simulink model "MODEL_BicycleModel_Integrator_SS_and_TF"  (R2019b)
settings: Solver=ode45  StartTime=0.0  StopTime=500  MaxStep=0.01  RelTol=1e-3  EnableMultiTasking=on
values from neighbouring files (symbols this model uses):
  a = vehicle(i).a    [SCRIPT_BicycleModel_Integrator_SS_and_TF.m]
  A = [(Caf+Car)/(m*U) (a*Caf-b*Car)/(m*U)-U ... (first row only)    [SCRIPT_BicycleModel_Integrator_SS_and_TF.m]
  b = vehicle(i).b    [SCRIPT_BicycleModel_Integrator_SS_and_TF.m]
  B = [-Caf/m -Car/m; -a*Caf/Iz b*Car/Iz]    [SCRIPT_BicycleModel_Integrator_SS_and_TF.m]
  Caf = vehicle(i).Caf    [SCRIPT_BicycleModel_Integrator_SS_and_TF.m]
  Car = vehicle(i).Car    [SCRIPT_BicycleModel_Integrator_SS_and_TF.m]
  den = [1 -((Caf+Car)/(m*U)+(Caf*a^2+Car*b^2)/(Iz*U)) (Caf*Car*L^2/(m*Iz*U^2)+(a*Caf-b*Car)/Iz)]    [SCRIPT_BicycleModel_Integrator_SS_and_TF.m]
  Iz = vehicle(i).Iz    [SCRIPT_BicycleModel_Integrator_SS_and_TF.m]
  m = vehicle(i).m    [SCRIPT_BicycleModel_Integrator_SS_and_TF.m]
  num_latvel = [-Caf/m b*Caf*Car*L/(m*U*Iz)+a*Caf*U/Iz]    [SCRIPT_BicycleModel_Integrator_SS_and_TF.m]
  num_yawrate = [-a*Caf/Iz Caf*Car*L/(m*U*Iz)]    [SCRIPT_BicycleModel_Integrator_SS_and_TF.m]
  U = 20    [SCRIPT_BicycleModel_Integrator_SS_and_TF.m]
settings Model: Creator=snb10  LastModifiedBy=Dada
settings DataIOCC: LimitDataPoints=on  SaveFormat=Array  SignalLoggingSaveFormat=ModelDataLogs  ReturnWorkspaceOutputs=off  SignalLoggingName=sigsOut
settings OptimizationCC: InitFltsAndDblsToZero=on  LifeSpan=inf
settings DebuggingCC: SaveWithParameterizedLinksMsg=none  UnderspecifiedInitializationDetection=Classic  MergeDetectMultiDrivingBlocksExec=none  SignalResolutionControl=TryResolveAllWithWarning  MultiTaskDSMMsg=warning  MultiTaskCondExecSysMsg=none  FcnCallInpInsideContextMsg=warning  StateNameClashWarn=warning  SFUnexpectedBacktrackingDiag=warning  SFNoUnconditionalDefaultTransitionDiag=warning  SFExecutionAtInitializationDiag=none  ArithmeticOperatorsInVariantConditions=warning
settings HardwareCC: ProdBitPerPointer=32  ProdBitPerSizeT=32  ProdBitPerPtrDiffT=32  ProdLargestAtomicFloat=None  ProdIntDivRoundTo=Undefined  ProdEndianess=Unspecified  ProdWordSize=32  ProdHWDeviceType=32-bit Generic  TargetUnknown=on
settings ModelReferenceCC: PropagateSignalLabelsOutOfModel=off
settings SFSimCC: SimUseLocalCustomCode=off  CustomCodeUndefinedFunction=UseInterfaceOnly
settings RTWCC: RTWUseLocalCustomCode=off
settings CodeAppCC: StateflowObjectComments=on
settings GRTTargetCC: TargetFcnLib=ansi_tfl_tmw.mat  TargetLangStandard=C89/C90 (ANSI)  GeneratePreprocessorConditionals=Disable all  CombineOutputUpdateFcns=off  GRTInterface=on
settings ConfigComp: CovMetricSettings=dw  CovHtmlReporting=on  CovSaveCumulativeToWorkspaceVar=on  CovSaveSingleToWorkspaceVar=on  CovExternalEMLEnable=off

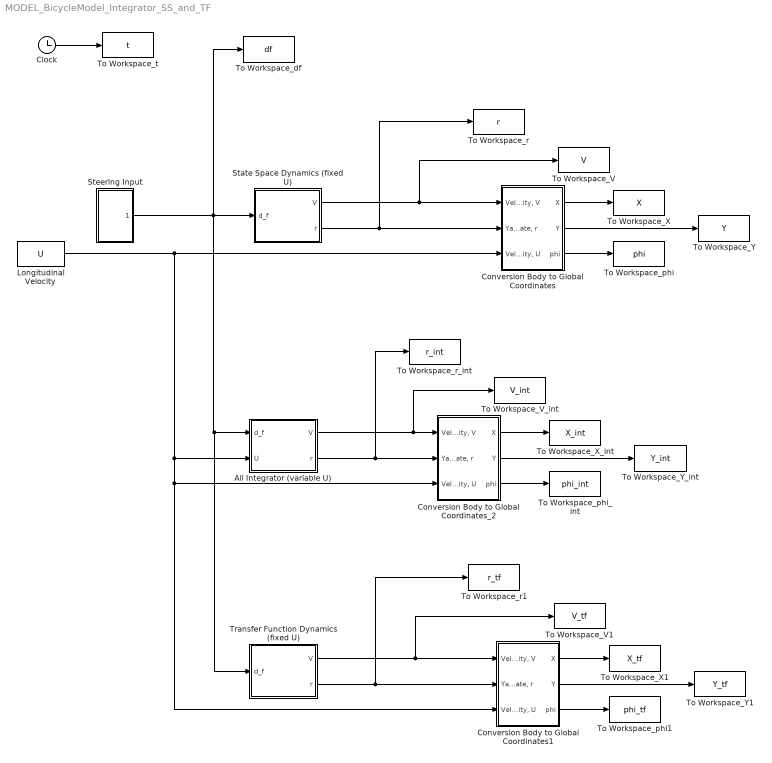
== system MODEL_BicycleModel_Integrator_SS_and_TF ==
  All Integrator (variable U) : Subsystem
  Clock : Clock
  Conversion Body to Global Coordinates : Subsystem
  Conversion Body to Global Coordinates1 : Subsystem
  Conversion Body to Global Coordinates_2 : Subsystem
  Longitudinal Velocity : Constant  Value=U
  State Space Dynamics (fixed U) : Subsystem
  Steering Input : Subsystem
  To Workspace_V : ToWorkspace  VariableName=V  SampleTime=-1
  To Workspace_V1 : ToWorkspace  VariableName=V_tf  SampleTime=-1
  To Workspace_V_int : ToWorkspace  VariableName=V_int  SampleTime=-1
  To Workspace_X : ToWorkspace  VariableName=X  SampleTime=-1
  To Workspace_X1 : ToWorkspace  VariableName=X_tf  SampleTime=-1
  To Workspace_X_int : ToWorkspace  VariableName=X_int  SampleTime=-1
  To Workspace_Y : ToWorkspace  VariableName=Y  SampleTime=-1
  To Workspace_Y1 : ToWorkspace  VariableName=Y_tf  SampleTime=-1
  To Workspace_Y_int : ToWorkspace  VariableName=Y_int  SampleTime=-1
  To Workspace_df : ToWorkspace  VariableName=df  SampleTime=-1
  To Workspace_phi : ToWorkspace  VariableName=phi  SampleTime=-1
  To Workspace_phi1 : ToWorkspace  VariableName=phi_tf  SampleTime=-1
  To Workspace_phi_int : ToWorkspace  VariableName=phi_int  SampleTime=-1
  To Workspace_r : ToWorkspace  VariableName=r  SampleTime=-1
  To Workspace_r1 : ToWorkspace  VariableName=r_tf  SampleTime=-1
  To Workspace_r_int : ToWorkspace  VariableName=r_int  SampleTime=-1
  To Workspace_t : ToWorkspace  VariableName=t  SampleTime=-1
  Transfer Function Dynamics (fixed U) : Subsystem
  wires:
  Conversion Body to Global Coordinates/1(X) -> To Workspace_X/1
  Conversion Body to Global Coordinates/2(Y) -> To Workspace_Y/1
  Conversion Body to Global Coordinates/3(phi) -> To Workspace_phi/1
  Clock/1 -> To Workspace_t/1
  All Integrator (variable U)/1(V) -> Conversion Body to Global Coordinates_2/1("Velocity, V"), To Workspace_V_int/1
  Conversion Body to Global Coordinates_2/1(X) -> To Workspace_X_int/1
  Conversion Body to Global Coordinates_2/2(Y) -> To Workspace_Y_int/1
  All Integrator (variable U)/2(r) -> Conversion Body to Global Coordinates_2/2("Yaw Rate, r"), To Workspace_r_int/1
  Conversion Body to Global Coordinates_2/3(phi) -> To Workspace_phi_int/1
  State Space Dynamics (fixed U)/1(V) -> To Workspace_V/1, Conversion Body to Global Coordinates/1("Velocity, V")
  State Space Dynamics (fixed U)/2(r) -> To Workspace_r/1, Conversion Body to Global Coordinates/2("Yaw Rate, r")
  Conversion Body to Global Coordinates1/1(X) -> To Workspace_X1/1
  Conversion Body to Global Coordinates1/2(Y) -> To Workspace_Y1/1
  Longitudinal Velocity/1 -> Conversion Body to Global Coordinates/3("Velocity, U"), Conversion Body to Global Coordinates1/3("Velocity, U"), Conversion Body to Global Coordinates_2/3("Velocity, U"), All Integrator (variable U)/2(U)
  Conversion Body to Global Coordinates1/3(phi) -> To Workspace_phi1/1
  Steering Input/1(delta_f) -> State Space Dynamics (fixed U)/1(d_f), To Workspace_df/1, Transfer Function Dynamics (fixed U)/1(d_f), All Integrator (variable U)/1(d_f)
  Transfer Function Dynamics (fixed U)/1(V) -> To Workspace_V1/1, Conversion Body to Global Coordinates1/1("Velocity, V")
  Transfer Function Dynamics (fixed U)/2(r) -> To Workspace_r1/1, Conversion Body to Global Coordinates1/2("Yaw Rate, r")

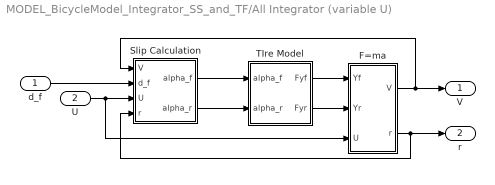
== system MODEL_BicycleModel_Integrator_SS_and_TF/All Integrator (variable U) ==
  d_f : Inport
  U : Inport  Port=2
  F=ma : Subsystem
  Slip Calculation : Subsystem
  TIre Model : Subsystem
  V : Outport
  r : Outport  Port=2
  wires:
  Slip Calculation/1(alpha_f) -> TIre Model/1(alpha_f)
  Slip Calculation/2(alpha_r) -> TIre Model/2(alpha_r)
  TIre Model/1(Fyf) -> F=ma/1(Yf)
  TIre Model/2(Fyr) -> F=ma/2(Yr)
  U/1 -> Slip Calculation/3(U), F=ma/3(" U")
  d_f/1 -> Slip Calculation/2(d_f)
  F=ma/1(V) -> V/1, Slip Calculation/1(V)
  F=ma/2(r) -> r/1, Slip Calculation/4(r)

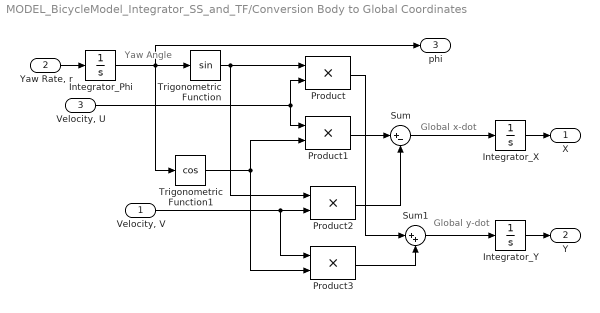
== system MODEL_BicycleModel_Integrator_SS_and_TF/Conversion Body to Global Coordinates ==
  note: Yaw Angle
  note: Global x-dot
  note: Global y-dot
  "Velocity, V" : Inport
  "Yaw Rate, r" : Inport  Port=2
  "Velocity, U" : Inport  Port=3
  Integrator_Phi : Integrator
  Integrator_X : Integrator
  Integrator_Y : Integrator
  Product{,1..3} (4 alike) : Product  SaturateOnIntegerOverflow=on  OutDataTypeStr=Inherit: Same as first input
  Sum : Sum  Inputs=|+-  SaturateOnIntegerOverflow=on
  Sum1 : Sum  Inputs=|++  SaturateOnIntegerOverflow=on
  Trigonometric Function : Trigonometry
  Trigonometric Function1 : Trigonometry  Operator=cos
  X : Outport
  Y : Outport  Port=2
  phi : Outport  Port=3
  wires:
  Integrator_Phi/1 -> Trigonometric Function/1, Trigonometric Function1/1, phi/1
  "Velocity, U"/1 -> Product/2, Product1/1
  "Velocity, V"/1 -> Product2/2, Product3/1
  Trigonometric Function1/1 -> Product1/2, Product3/2
  Product1/1 -> Sum/1
  Product2/1 -> Sum/2
  Trigonometric Function/1 -> Product/1, Product2/1
  Sum/1 -> Integrator_X/1
  Product/1 -> Sum1/1
  Product3/1 -> Sum1/2
  Sum1/1 -> Integrator_Y/1
  "Yaw Rate, r"/1 -> Integrator_Phi/1
  Integrator_X/1 -> X/1
  Integrator_Y/1 -> Y/1

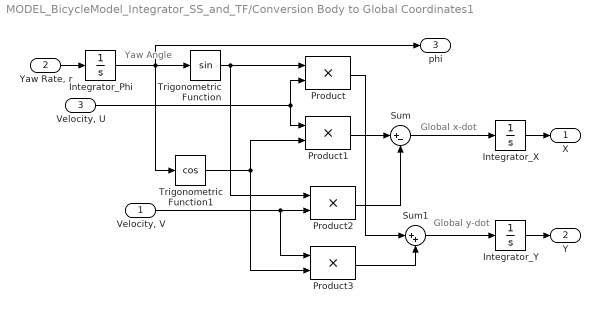
== system MODEL_BicycleModel_Integrator_SS_and_TF/Conversion Body to Global Coordinates1 ==
  note: Yaw Angle
  note: Global x-dot
  note: Global y-dot
  "Velocity, V" : Inport
  "Yaw Rate, r" : Inport  Port=2
  "Velocity, U" : Inport  Port=3
  Integrator_Phi : Integrator
  Integrator_X : Integrator
  Integrator_Y : Integrator
  Product{,1..3} (4 alike) : Product  SaturateOnIntegerOverflow=on  OutDataTypeStr=Inherit: Same as first input
  Sum : Sum  Inputs=|+-  SaturateOnIntegerOverflow=on
  Sum1 : Sum  Inputs=|++  SaturateOnIntegerOverflow=on
  Trigonometric Function : Trigonometry
  Trigonometric Function1 : Trigonometry  Operator=cos
  X : Outport
  Y : Outport  Port=2
  phi : Outport  Port=3
  wires:
  Integrator_Phi/1 -> Trigonometric Function/1, Trigonometric Function1/1, phi/1
  "Velocity, U"/1 -> Product/2, Product1/1
  "Velocity, V"/1 -> Product2/2, Product3/1
  Trigonometric Function1/1 -> Product1/2, Product3/2
  Product1/1 -> Sum/1
  Product2/1 -> Sum/2
  Trigonometric Function/1 -> Product/1, Product2/1
  Sum/1 -> Integrator_X/1
  Product/1 -> Sum1/1
  Product3/1 -> Sum1/2
  Sum1/1 -> Integrator_Y/1
  "Yaw Rate, r"/1 -> Integrator_Phi/1
  Integrator_X/1 -> X/1
  Integrator_Y/1 -> Y/1

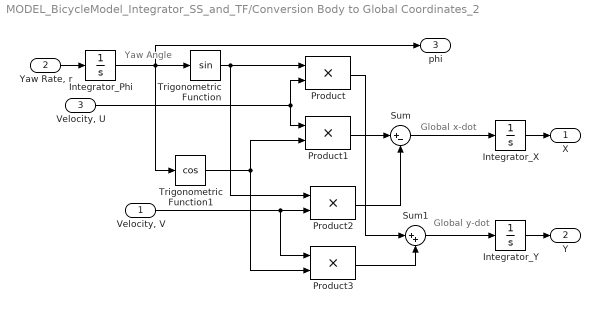
== system MODEL_BicycleModel_Integrator_SS_and_TF/Conversion Body to Global Coordinates_2 ==
  note: Global y-dot
  note: Global x-dot
  note: Yaw Angle
  "Velocity, V" : Inport
  "Yaw Rate, r" : Inport  Port=2
  "Velocity, U" : Inport  Port=3
  Integrator_Phi : Integrator
  Integrator_X : Integrator
  Integrator_Y : Integrator
  Product{,1..3} (4 alike) : Product  SaturateOnIntegerOverflow=on  OutDataTypeStr=Inherit: Same as first input
  Sum : Sum  Inputs=|+-  SaturateOnIntegerOverflow=on
  Sum1 : Sum  Inputs=|++  SaturateOnIntegerOverflow=on
  Trigonometric Function : Trigonometry
  Trigonometric Function1 : Trigonometry  Operator=cos
  X : Outport
  Y : Outport  Port=2
  phi : Outport  Port=3
  wires:
  Integrator_Y/1 -> Y/1
  Integrator_X/1 -> X/1
  "Yaw Rate, r"/1 -> Integrator_Phi/1
  Sum1/1 -> Integrator_Y/1
  Product3/1 -> Sum1/2
  Product/1 -> Sum1/1
  Sum/1 -> Integrator_X/1
  Trigonometric Function/1 -> Product2/1, Product/1
  Product2/1 -> Sum/2
  Product1/1 -> Sum/1
  Trigonometric Function1/1 -> Product3/2, Product1/2
  "Velocity, V"/1 -> Product3/1, Product2/2
  "Velocity, U"/1 -> Product1/1, Product/2
  Integrator_Phi/1 -> phi/1, Trigonometric Function1/1, Trigonometric Function/1

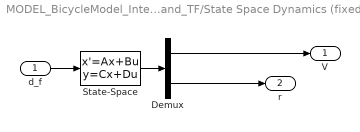
== system MODEL_BicycleModel_Integrator_SS_and_TF/State Space Dynamics (fixed U) ==
  d_f : Inport
  Demux : Demux  Outputs=2
  State-Space : StateSpace  A=A  B=B(:,1)  C=eye(2)  D=zeros(2,1)  InitialCondition=0
  V : Outport
  r : Outport  Port=2
  wires:
  State-Space/1 -> Demux/1
  Demux/1 -> V/1
  Demux/2 -> r/1
  d_f/1 -> State-Space/1

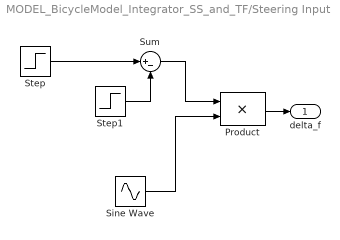
== system MODEL_BicycleModel_Integrator_SS_and_TF/Steering Input ==
  Product : Product  SaturateOnIntegerOverflow=on  OutDataTypeStr=Inherit: Same as first input
  Sine Wave : Sin  Amplitude=2*pi/180  Frequency=0.01*2*pi  SampleTime=0
  Step : Step  Time=0  SampleTime=0
  Step1 : Step  Time=100  SampleTime=0
  Sum : Sum  Inputs=|+-  SaturateOnIntegerOverflow=on
  delta_f : Outport
  wires:
  Step/1 -> Sum/1
  Step1/1 -> Sum/2
  Sum/1 -> Product/1
  Sine Wave/1 -> Product/2
  Product/1 -> delta_f/1

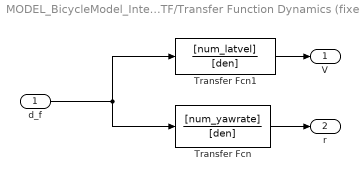
== system MODEL_BicycleModel_Integrator_SS_and_TF/Transfer Function Dynamics (fixed U) ==
  d_f : Inport
  Transfer Fcn : TransferFcn  Numerator=[num_yawrate]  Denominator=[den]
  Transfer Fcn1 : TransferFcn  Numerator=[num_latvel]  Denominator=[den]
  V : Outport
  r : Outport  Port=2
  wires:
  d_f/1 -> Transfer Fcn1/1, Transfer Fcn/1
  Transfer Fcn/1 -> r/1
  Transfer Fcn1/1 -> V/1

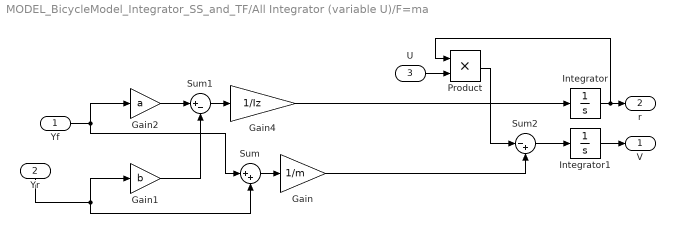
== system MODEL_BicycleModel_Integrator_SS_and_TF/All Integrator (variable U)/F=ma ==
  Yf : Inport
  Yr : Inport  Port=2
  " U" : Inport  Port=3
  Gain : Gain  Gain=1/m
  Gain1 : Gain  Gain=b
  Gain2 : Gain  Gain=a
  Gain4 : Gain  Gain=1/Iz
  Integrator : Integrator
  Integrator1 : Integrator
  Product : Product  RndMeth=Zero
  Sum : Sum  Inputs=|++
  Sum1 : Sum  Inputs=|+-
  Sum2 : Sum  Inputs=|-+
  V : Outport
  r : Outport  Port=2
  wires:
  Yf/1 -> Sum/1, Gain2/1
  Yr/1 -> Gain1/1, Sum/2
  Gain2/1 -> Sum1/1
  Gain1/1 -> Sum1/2
  Sum1/1 -> Gain4/1
  Gain4/1 -> Integrator/1
  Sum/1 -> Gain/1
  Product/1 -> Sum2/1
  Gain/1 -> Sum2/2
  Sum2/1 -> Integrator1/1
  Integrator/1 -> r/1, Product/1
  Integrator1/1 -> V/1
  " U"/1 -> Product/2

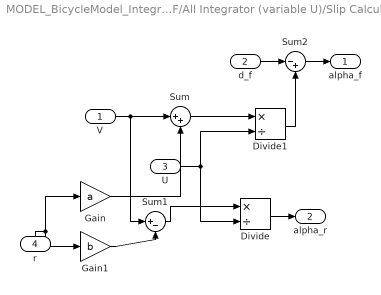
== system MODEL_BicycleModel_Integrator_SS_and_TF/All Integrator (variable U)/Slip Calculation ==
  V : Inport
  d_f : Inport  Port=2
  U : Inport  Port=3
  r : Inport  Port=4
  Divide : Product  Inputs=*/
  Divide1 : Product  Inputs=*/
  Gain : Gain  Gain=a
  Gain1 : Gain  Gain=b
  Sum : Sum  Inputs=|++
  Sum1 : Sum  Inputs=|+-
  Sum2 : Sum  Inputs=|-+
  alpha_f : Outport
  alpha_r : Outport  Port=2
  wires:
  V/1 -> Sum/1, Sum1/1
  Gain/1 -> Sum/2
  r/1 -> Gain/1, Gain1/1
  Gain1/1 -> Sum1/2
  Sum/1 -> Divide1/1
  U/1 -> Divide/2, Divide1/2
  Sum1/1 -> Divide/1
  Divide1/1 -> Sum2/2
  d_f/1 -> Sum2/1
  Sum2/1 -> alpha_f/1
  Divide/1 -> alpha_r/1

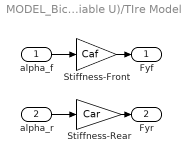
== system MODEL_BicycleModel_Integrator_SS_and_TF/All Integrator (variable U)/TIre Model ==
  alpha_f : Inport
  alpha_r : Inport  Port=2
  Stiffness-Front : Gain  Gain=Caf
  Stiffness-Rear : Gain  Gain=Car
  Fyf : Outport
  Fyr : Outport  Port=2
  wires:
  alpha_f/1 -> Stiffness-Front/1
  Stiffness-Front/1 -> Fyf/1
  alpha_r/1 -> Stiffness-Rear/1
  Stiffness-Rear/1 -> Fyr/1
